simulink library "csc_spc_sensor_processing_mtv_lib"  (R2014b)
settings: Solver=ode45  StartTime=0.0  StopTime=10.0  RelTol=1e-3
undefined symbols (not defined in the file or in its folder): kfl_use_mems
libraries: util_info_lib x1, csu_imp_imager_messsage_processing_lib x1, csu_lmp_lidar_messsage_processing_lib x1, csu_mmp_mems_messsage_processing_lib x1, csu_pgp_piksi_gps_processing_lib x1, csu_smp_sensonor_messsage_processing_lib x1, csu_tmp_tracker_messsage_processing_lib x1
settings Model: Creator=escrane  LastModifiedBy=mstewart

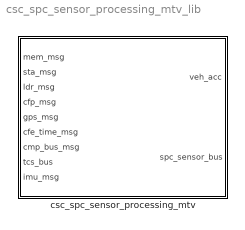
== system csc_spc_sensor_processing_mtv_lib ==
  csc_spc_sensor_processing_mtv : Subsystem

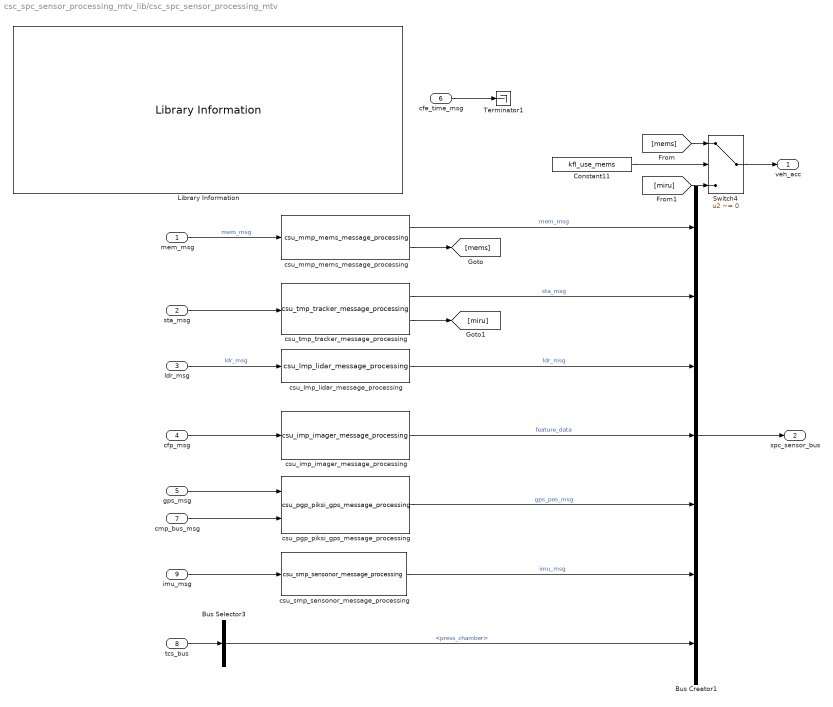
== system csc_spc_sensor_processing_mtv_lib/csc_spc_sensor_processing_mtv ==
  mem_msg : Inport
  sta_msg : Inport  Port=2
  ldr_msg : Inport  Port=3
  cfp_msg : Inport  Port=4
  gps_msg : Inport  Port=5
  cfe_time_msg : Inport  Port=6
  cmp_bus_msg : Inport  Port=7
  tcs_bus : Inport  Port=8
  imu_msg : Inport  Port=9
  Bus Creator1 : BusCreator  Inputs=7
  Bus Selector3 : BusSelector  OutputSignals=converted_pressures.press_chamber
  Constant11 : Constant  Value=kfl_use_mems
  Library Information : util_info_lib/Library Information  owner='escrane'
  Switch4 : Switch  Criteria=u2 ~= 0
  Terminator1 : Terminator
  csu_imp_imager_message_processing : csu_imp_imager_messsage_processing_lib/csu_imp_imager_message_processing
  csu_lmp_lidar_message_processing : csu_lmp_lidar_messsage_processing_lib/csu_lmp_lidar_message_processing
  csu_mmp_mems_message_processing : csu_mmp_mems_messsage_processing_lib/csu_mmp_mems_message_processing
  csu_pgp_piksi_gps_message_processing : csu_pgp_piksi_gps_processing_lib/csu_pgp_piksi_gps_message_processing
  csu_smp_sensonor_message_processing : csu_smp_sensonor_messsage_processing_lib/csu_smp_sensonor_message_processing
  csu_tmp_tracker_message_processing : csu_tmp_tracker_messsage_processing_lib/csu_tmp_tracker_message_processing
  veh_acc : Outport
  spc_sensor_bus : Outport  Port=2
  wires:
  csu_smp_sensonor_message_processing/1 -> Bus Creator1/6  "imu_msg"
  imu_msg/1 -> csu_smp_sensonor_message_processing/1
  Bus Selector3/1 -> Bus Creator1/7  "<press_chamber>"
  tcs_bus/1 -> Bus Selector3/1
  csu_pgp_piksi_gps_message_processing/1 -> Bus Creator1/5  "gps_pos_msg"
  gps_msg/1 -> csu_pgp_piksi_gps_message_processing/1
  Switch4/1 -> veh_acc/1
  Constant11/1 -> Switch4/2
  csu_lmp_lidar_message_processing/1 -> Bus Creator1/3  "ldr_msg"
  cfe_time_msg/1 -> Terminator1/1
  cmp_bus_msg/1 -> csu_pgp_piksi_gps_message_processing/2
  Bus Creator1/1 -> spc_sensor_bus/1
  sta_msg/1 -> csu_tmp_tracker_message_processing/1
  mem_msg/1 -> csu_mmp_mems_message_processing/1  "mem_msg"
  ldr_msg/1 -> csu_lmp_lidar_message_processing/1  "ldr_msg"
  cfp_msg/1 -> csu_imp_imager_message_processing/1
  csu_tmp_tracker_message_processing/1 -> Bus Creator1/2  "sta_msg"
  csu_mmp_mems_message_processing/1 -> Bus Creator1/1  "mem_msg"
  csu_imp_imager_message_processing/1 -> Bus Creator1/4  "feature_data"
  csu_mmp_mems_message_processing/2 -> [mems]
  [mems] -> Switch4/1
  csu_tmp_tracker_message_processing/2 -> [miru]
  [miru] -> Switch4/3
